simulink model "ADANISS_2R_Control"  (R2025b)
settings: Solver=ode45  StartTime=0  StopTime=40  MaxStep=0.0005  MinStep=1e-6  RelTol=1e-5  AbsTol=1e-7
libraries: slpidlib x2
settings Model: Creator=nicao  LastModifiedBy=nicao

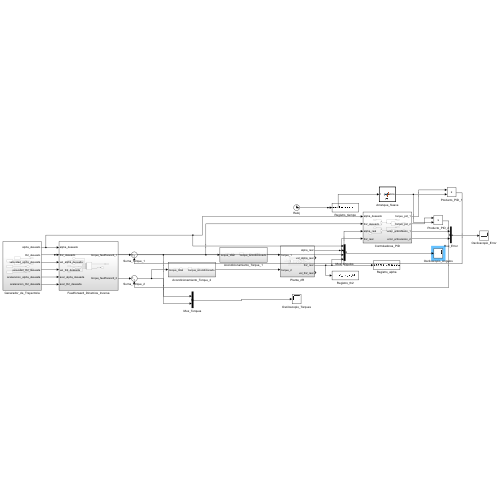
[thumbnail: Simulink's stored preview of the top-level diagram]
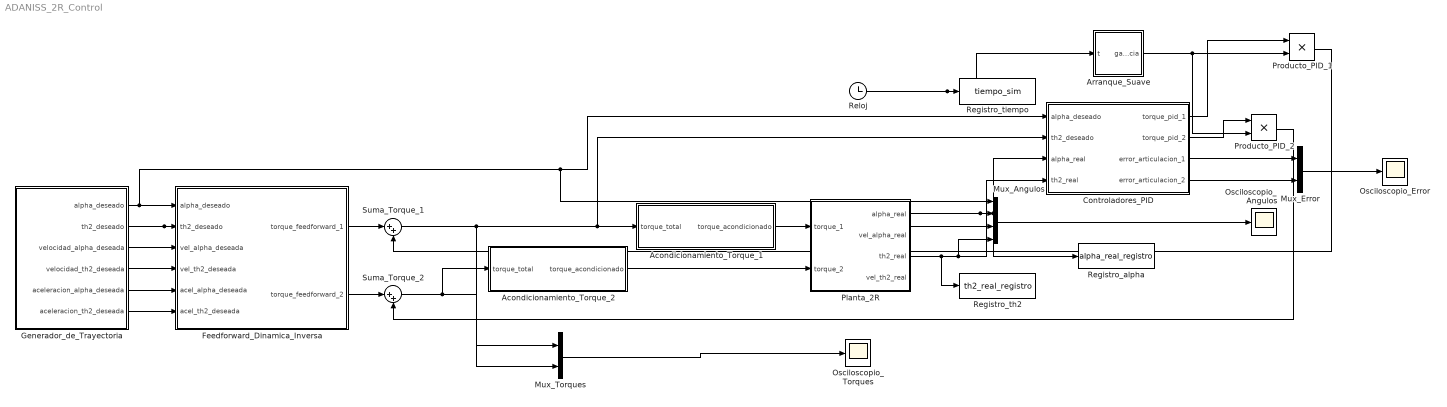
== system ADANISS_2R_Control ==
  Acondicionamiento_Torque_1 : Subsystem
  Acondicionamiento_Torque_2 : Subsystem
  Arranque_Suave : MATLAB Function  TreatAsAtomicUnit=on
  Controladores_PID : Subsystem
  Feedforward_Dinamica_Inversa : Subsystem
  Generador_de_Trayectoria : Subsystem
  Mux_Angulos : Mux
  Mux_Error : Mux  Inputs=2
  Mux_Torques : Mux  Inputs=2
  Osciloscopio_Angulos : Scope
      settings: ActiveDisplayYMinimum=-15.541303883024996  ActiveDisplayYMaximum=18.854538421738404
  Osciloscopio_Error : Scope
      settings: ActiveDisplayYMinimum=-0.62688226999815022  ActiveDisplayYMaximum=1.0560129058216277
  Osciloscopio_Torques : Scope
      settings: ActiveDisplayYMinimum=-3.9250000000000003  ActiveDisplayYMaximum=3.9250000000000003
  Planta_2R : Subsystem
  Producto_PID_1 : Product
  Producto_PID_2 : Product
  Registro_alpha : ToWorkspace  VariableName=alpha_real_registro
  Registro_th2 : ToWorkspace  VariableName=th2_real_registro
  Registro_tiempo : ToWorkspace  VariableName=tiempo_sim
  Reloj : Clock
  Suma_Torque_1 : Sum  Inputs=|++
  Suma_Torque_2 : Sum  Inputs=|++
  wires:
  Generador_de_Trayectoria/1(alpha_deseado) -> Mux_Angulos/1, Controladores_PID/1(alpha_deseado), Feedforward_Dinamica_Inversa/1(alpha_deseado)
  Generador_de_Trayectoria/2(th2_deseado) -> Mux_Angulos/3, Controladores_PID/2(th2_deseado), Feedforward_Dinamica_Inversa/2(th2_deseado)
  Generador_de_Trayectoria/3(velocidad_alpha_deseada) -> Feedforward_Dinamica_Inversa/3(vel_alpha_deseada)
  Generador_de_Trayectoria/4(velocidad_th2_deseada) -> Feedforward_Dinamica_Inversa/4(vel_th2_deseada)
  Generador_de_Trayectoria/5(aceleracion_alpha_deseada) -> Feedforward_Dinamica_Inversa/5(acel_alpha_deseada)
  Generador_de_Trayectoria/6(aceleracion_th2_deseada) -> Feedforward_Dinamica_Inversa/6(acel_th2_deseada)
  Planta_2R/1(alpha_real) -> Registro_alpha/1, Controladores_PID/3(alpha_real), Mux_Angulos/2
  Planta_2R/3(th2_real) -> Registro_th2/1, Mux_Angulos/4, Controladores_PID/4(th2_real)
  Suma_Torque_1/1 -> Mux_Torques/1, Acondicionamiento_Torque_1/1(torque_total)
  Suma_Torque_2/1 -> Acondicionamiento_Torque_2/1(torque_total), Mux_Torques/2
  Acondicionamiento_Torque_1/1(torque_acondicionado) -> Planta_2R/1(torque_1)
  Acondicionamiento_Torque_2/1(torque_acondicionado) -> Planta_2R/2(torque_2)
  Mux_Angulos/1 -> Osciloscopio_Angulos/1
  Mux_Torques/1 -> Osciloscopio_Torques/1
  Controladores_PID/3(error_articulacion_1) -> Mux_Error/1
  Controladores_PID/4(error_articulacion_2) -> Mux_Error/2
  Mux_Error/1 -> Osciloscopio_Error/1
  Reloj/1 -> Arranque_Suave/1(t), Registro_tiempo/1
  Arranque_Suave/1(ganancia) -> Producto_PID_2/2, Producto_PID_1/2
  Controladores_PID/1(torque_pid_1) -> Producto_PID_1/1
  Producto_PID_1/1 -> Suma_Torque_1/2
  Controladores_PID/2(torque_pid_2) -> Producto_PID_2/1
  Producto_PID_2/1 -> Suma_Torque_2/2
  Feedforward_Dinamica_Inversa/1(torque_feedforward_1) -> Suma_Torque_1/1
  Feedforward_Dinamica_Inversa/2(torque_feedforward_2) -> Suma_Torque_2/1

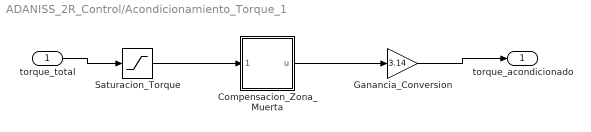
== system ADANISS_2R_Control/Acondicionamiento_Torque_1 ==
  torque_total : Inport
  Compensacion_Zona_Muerta : MATLAB Function  TreatAsAtomicUnit=on
  Ganancia_Conversion : Gain  Gain=3.14
  Saturacion_Torque : Saturate  UpperLimit=3.14  LowerLimit=-3.14
  torque_acondicionado : Outport
  wires:
  Saturacion_Torque/1 -> Compensacion_Zona_Muerta/1(tau_sat)
  Compensacion_Zona_Muerta/1(u) -> Ganancia_Conversion/1
  torque_total/1 -> Saturacion_Torque/1
  Ganancia_Conversion/1 -> torque_acondicionado/1

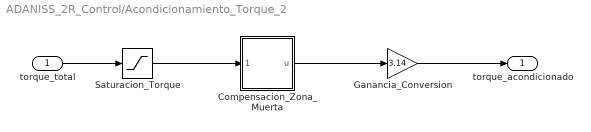
== system ADANISS_2R_Control/Acondicionamiento_Torque_2 ==
  torque_total : Inport
  Compensacion_Zona_Muerta : MATLAB Function  TreatAsAtomicUnit=on
  Ganancia_Conversion : Gain  Gain=3.14
  Saturacion_Torque : Saturate  UpperLimit=3.14  LowerLimit=-3.14
  torque_acondicionado : Outport
  wires:
  torque_total/1 -> Saturacion_Torque/1
  Saturacion_Torque/1 -> Compensacion_Zona_Muerta/1(tau_sat)
  Compensacion_Zona_Muerta/1(u) -> Ganancia_Conversion/1
  Ganancia_Conversion/1 -> torque_acondicionado/1

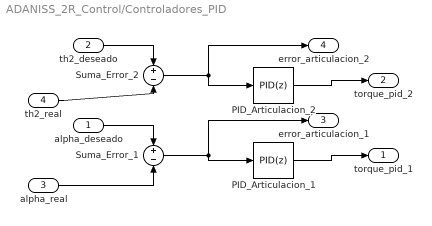
== system ADANISS_2R_Control/Controladores_PID ==
  alpha_deseado : Inport
  th2_deseado : Inport  Port=2
  alpha_real : Inport  Port=3
  th2_real : Inport  Port=4
  PID_Articulacion_1 : slpidlib/PID Controller  Controller=PID  Form=Parallel  TimeDomain=Discrete-time  UseExternalTs=off  SampleTime=0.001  IntegratorMethod=Forward Euler  FilterMethod=Forward Euler  ControllerParametersSource=internal  P=15  I=8  UseKiTs=off  D=1.2  UseExternalDerivativeSource=off  N=50  UseFilter=on  TunerSelectOption=Transfer Function Based (PID Tuner App)  InitialConditionSource=internal  InitialConditionForIntegrator=0  InitialConditionForFilter=0  DifferentiatorICPrevScaledInput=0  ExternalReset=none  TrackingMode=off  Kt=1  LimitOutput=on  SatLimitsSource=internal  UpperSaturationLimit=3.14  LowerSaturationLimit=-3.14  LinearizeAsGain=on  AntiWindupMode=clamping  Kb=1  LimitIntegrator=off  UpperIntegratorSaturationLimit=inf  LowerIntegratorSaturationLimit=-inf  POutMin=[]  POutMax=[]  IOutMin=[]  IOutMax=[]  DOutMin=[]  DOutMax=[]  NOutMin=[]  NOutMax=[]  SumOutMin=[]  SumOutMax=[]  SaturationOutMin=[]  SaturationOutMax=[]  PParamMin=[]  PParamMax=[]  IParamMin=[]  IParamMax=[]  DParamMin=[]  DParamMax=[]  NParamMin=[]  NParamMax=[]  KbParamMin=[]  KbParamMax=[]  KtParamMin=[]  KtParamMax=[]  KbOutMin=[]  KbOutMax=[]  KtOutMin=[]  KtOutMax=[]  IntegratorOutMin=[]  IntegratorOutMax=[]  FilterOutMin=[]  FilterOutMax=[]  SumI1OutMin=[]  SumI1OutMax=[]  SumI2OutMin=[]  SumI2OutMax=[]  SumI3OutMin=[]  SumI3OutMax=[]  SumI4OutMin=[]  SumI4OutMax=[]  SumDOutMin=[]  SumDOutMax=[]  DifferentiatorOutMin=[]  DifferentiatorOutMax=[]  FilterDiffOutCoefMin=[]  FilterDiffOutCoefMax=[]  ReciprocalOutMin=[]  ReciprocalOutMax=[]  SumDenOutMin=[]  SumDenOutMax=[]  SumNumOutMin=[]  SumNumOutMax=[]  DivideOutMin=[]  DivideOutMax=[]  UdiffTsProdOutMin=[]  UdiffTsProdOutMax=[]  NTsProdOutMin=[]  NTsProdOutMax=[]  UintegralTsProdOutMin=[]  UintegralTsProdOutMax=[]  UngainTsProdOutMin=[]  UngainTsProdOutMax=[]  ClampingZeroOutDataTypeStr=Inherit: Inherit via back propagation  ClampingZeroOutMin=[]  ClampingZeroOutMax=[]  FilterDenConstantOutDataTypeStr=Inherit: Inherit via back propagation  FilterDenConstantOutMin=[]  FilterDenConstantOutMax=[]  PCopyOutDataTypeStr=Inherit: Inherit via back propagation  PCopyOutMin=[]  PCopyOutMax=[]  NCopyOutDataTypeStr=Inherit: Inherit via back propagation  NCopyOutMin=[]  NCopyOutMax=[]  IntegratorContinuousStateAttributes=''  IntegratorStateMustResolveToSignalObject=off  IntegratorRTWStateStorageClass=Auto  FilterContinuousStateAttributes=''  FilterStateMustResolveToSignalObject=off  FilterRTWStateStorageClass=Auto  ParallelPVariant=InternalParameters  IdealPVariant=Disabled  IVariant=InternalParameters  DVariant=InternalParameters  IntegratorVariant=Discrete  SatVariant=Enabled  AWVariant=DiscClampingParallel  PCopyVariant=Disabled  TRVariant=Disabled  FdbkBlocksVariant=Forward  IdealPFdbkVariant=Disabled  SatFdbkVariant=Disabled  DerivativeFilterVariant=ForwardEulerFilter  NVariant=InternalParameters  NCopyVariant=Disabled  FilterICVariant=InternalICsFilter  IntegratorICVariant=InternalICs  ExternalResetVariant=Disabled  TRSumVariant=Passthrough  SumFdbkVariant=Disabled  SumVariant=Sum_PID  TsampFilterVariant=InternalTs  TsampNgainVariant=Passthrough  TsampIntegralVariant=Disabled_SignalSpec  ExternalSaturationOutDataTypeStr=Inherit: Same as second input  DerivativeSourceVariant=ErrorSignal  PreIntVariant=InternalPreInt
  PID_Articulacion_2 : slpidlib/PID Controller  Controller=PID  Form=Parallel  TimeDomain=Discrete-time  UseExternalTs=off  SampleTime=0.001  IntegratorMethod=Forward Euler  FilterMethod=Forward Euler  ControllerParametersSource=internal  P=15  I=8  UseKiTs=off  D=1.2  UseExternalDerivativeSource=off  N=50  UseFilter=on  TunerSelectOption=Transfer Function Based (PID Tuner App)  InitialConditionSource=internal  InitialConditionForIntegrator=0  InitialConditionForFilter=0  DifferentiatorICPrevScaledInput=0  ExternalReset=none  TrackingMode=off  Kt=1  LimitOutput=on  SatLimitsSource=internal  UpperSaturationLimit=3.14  LowerSaturationLimit=-3.14  LinearizeAsGain=on  AntiWindupMode=clamping  Kb=1  LimitIntegrator=off  UpperIntegratorSaturationLimit=inf  LowerIntegratorSaturationLimit=-inf  POutMin=[]  POutMax=[]  IOutMin=[]  IOutMax=[]  DOutMin=[]  DOutMax=[]  NOutMin=[]  NOutMax=[]  SumOutMin=[]  SumOutMax=[]  SaturationOutMin=[]  SaturationOutMax=[]  PParamMin=[]  PParamMax=[]  IParamMin=[]  IParamMax=[]  DParamMin=[]  DParamMax=[]  NParamMin=[]  NParamMax=[]  KbParamMin=[]  KbParamMax=[]  KtParamMin=[]  KtParamMax=[]  KbOutMin=[]  KbOutMax=[]  KtOutMin=[]  KtOutMax=[]  IntegratorOutMin=[]  IntegratorOutMax=[]  FilterOutMin=[]  FilterOutMax=[]  SumI1OutMin=[]  SumI1OutMax=[]  SumI2OutMin=[]  SumI2OutMax=[]  SumI3OutMin=[]  SumI3OutMax=[]  SumI4OutMin=[]  SumI4OutMax=[]  SumDOutMin=[]  SumDOutMax=[]  DifferentiatorOutMin=[]  DifferentiatorOutMax=[]  FilterDiffOutCoefMin=[]  FilterDiffOutCoefMax=[]  ReciprocalOutMin=[]  ReciprocalOutMax=[]  SumDenOutMin=[]  SumDenOutMax=[]  SumNumOutMin=[]  SumNumOutMax=[]  DivideOutMin=[]  DivideOutMax=[]  UdiffTsProdOutMin=[]  UdiffTsProdOutMax=[]  NTsProdOutMin=[]  NTsProdOutMax=[]  UintegralTsProdOutMin=[]  UintegralTsProdOutMax=[]  UngainTsProdOutMin=[]  UngainTsProdOutMax=[]  ClampingZeroOutDataTypeStr=Inherit: Inherit via back propagation  ClampingZeroOutMin=[]  ClampingZeroOutMax=[]  FilterDenConstantOutDataTypeStr=Inherit: Inherit via back propagation  FilterDenConstantOutMin=[]  FilterDenConstantOutMax=[]  PCopyOutDataTypeStr=Inherit: Inherit via back propagation  PCopyOutMin=[]  PCopyOutMax=[]  NCopyOutDataTypeStr=Inherit: Inherit via back propagation  NCopyOutMin=[]  NCopyOutMax=[]  IntegratorContinuousStateAttributes=''  IntegratorStateMustResolveToSignalObject=off  IntegratorRTWStateStorageClass=Auto  FilterContinuousStateAttributes=''  FilterStateMustResolveToSignalObject=off  FilterRTWStateStorageClass=Auto  ParallelPVariant=InternalParameters  IdealPVariant=Disabled  IVariant=InternalParameters  DVariant=InternalParameters  IntegratorVariant=Discrete  SatVariant=Enabled  AWVariant=DiscClampingParallel  PCopyVariant=Disabled  TRVariant=Disabled  FdbkBlocksVariant=Forward  IdealPFdbkVariant=Disabled  SatFdbkVariant=Disabled  DerivativeFilterVariant=ForwardEulerFilter  NVariant=InternalParameters  NCopyVariant=Disabled  FilterICVariant=InternalICsFilter  IntegratorICVariant=InternalICs  ExternalResetVariant=Disabled  TRSumVariant=Passthrough  SumFdbkVariant=Disabled  SumVariant=Sum_PID  TsampFilterVariant=InternalTs  TsampNgainVariant=Passthrough  TsampIntegralVariant=Disabled_SignalSpec  ExternalSaturationOutDataTypeStr=Inherit: Same as second input  DerivativeSourceVariant=ErrorSignal  PreIntVariant=InternalPreInt
  Suma_Error_1 : Sum  Inputs=+-
  Suma_Error_2 : Sum  Inputs=+-
  torque_pid_1 : Outport
  torque_pid_2 : Outport  Port=2
  error_articulacion_1 : Outport  Port=3
  error_articulacion_2 : Outport  Port=4
  wires:
  alpha_deseado/1 -> Suma_Error_1/1
  alpha_real/1 -> Suma_Error_1/2
  th2_deseado/1 -> Suma_Error_2/1
  th2_real/1 -> Suma_Error_2/2
  Suma_Error_1/1 -> PID_Articulacion_1/1, error_articulacion_1/1
  Suma_Error_2/1 -> PID_Articulacion_2/1, error_articulacion_2/1
  PID_Articulacion_1/1 -> torque_pid_1/1
  PID_Articulacion_2/1 -> torque_pid_2/1

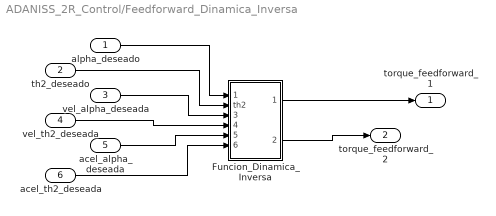
== system ADANISS_2R_Control/Feedforward_Dinamica_Inversa ==
  alpha_deseado : Inport
  th2_deseado : Inport  Port=2
  vel_alpha_deseada : Inport  Port=3
  vel_th2_deseada : Inport  Port=4
  acel_alpha_deseada : Inport  Port=5
  acel_th2_deseada : Inport  Port=6
  Funcion_Dinamica_Inversa : MATLAB Function  TreatAsAtomicUnit=on
  torque_feedforward_1 : Outport
  torque_feedforward_2 : Outport  Port=2
  wires:
  alpha_deseado/1 -> Funcion_Dinamica_Inversa/1(alpha)
  Funcion_Dinamica_Inversa/1(tau_ff1) -> torque_feedforward_1/1
  th2_deseado/1 -> Funcion_Dinamica_Inversa/2(th2)
  vel_alpha_deseada/1 -> Funcion_Dinamica_Inversa/3(dalpha)
  vel_th2_deseada/1 -> Funcion_Dinamica_Inversa/4(dth2)
  acel_alpha_deseada/1 -> Funcion_Dinamica_Inversa/5(d2alpha)
  acel_th2_deseada/1 -> Funcion_Dinamica_Inversa/6(d2th2)
  Funcion_Dinamica_Inversa/2(tau_ff2) -> torque_feedforward_2/1

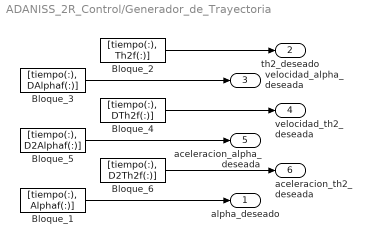
== system ADANISS_2R_Control/Generador_de_Trayectoria ==
  Bloque_1 : FromWorkspace  VariableName=[tiempo(:), Alphaf(:)]
  Bloque_2 : FromWorkspace  VariableName=[tiempo(:), Th2f(:)]
  Bloque_3 : FromWorkspace  VariableName=[tiempo(:), DAlphaf(:)]
  Bloque_4 : FromWorkspace  VariableName=[tiempo(:), DTh2f(:)]
  Bloque_5 : FromWorkspace  VariableName=[tiempo(:), D2Alphaf(:)]
  Bloque_6 : FromWorkspace  VariableName=[tiempo(:), D2Th2f(:)]
  alpha_deseado : Outport
  th2_deseado : Outport  Port=2
  velocidad_alpha_deseada : Outport  Port=3
  velocidad_th2_deseada : Outport  Port=4
  aceleracion_alpha_deseada : Outport  Port=5
  aceleracion_th2_deseada : Outport  Port=6
  wires:
  Bloque_1/1 -> alpha_deseado/1
  Bloque_2/1 -> th2_deseado/1
  Bloque_3/1 -> velocidad_alpha_deseada/1
  Bloque_4/1 -> velocidad_th2_deseada/1
  Bloque_5/1 -> aceleracion_alpha_deseada/1
  Bloque_6/1 -> aceleracion_th2_deseada/1

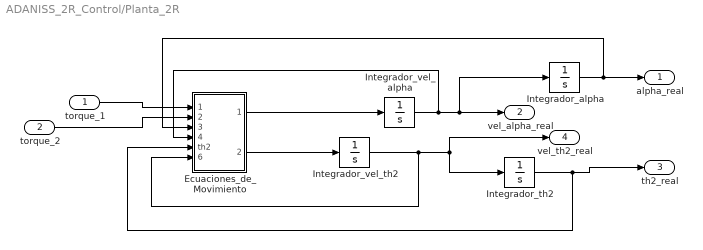
== system ADANISS_2R_Control/Planta_2R ==
  torque_1 : Inport
  torque_2 : Inport  Port=2
  Ecuaciones_de_Movimiento : MATLAB Function  TreatAsAtomicUnit=on
  Integrador_alpha : Integrator
  Integrador_th2 : Integrator  InitialCondition=3.141592653589793
  Integrador_vel_alpha : Integrator  InitialCondition=0.0004502450016226697
  Integrador_vel_th2 : Integrator  InitialCondition=-0.0003575475012871365
  alpha_real : Outport
  vel_alpha_real : Outport  Port=2
  th2_real : Outport  Port=3
  vel_th2_real : Outport  Port=4
  wires:
  torque_1/1 -> Ecuaciones_de_Movimiento/1(tau1)
  Ecuaciones_de_Movimiento/1(ddq1) -> Integrador_vel_alpha/1
  Integrador_vel_alpha/1 -> vel_alpha_real/1, Integrador_alpha/1, Ecuaciones_de_Movimiento/4(dalpha)
  Integrador_vel_th2/1 -> vel_th2_real/1, Integrador_th2/1, Ecuaciones_de_Movimiento/6(dth2)
  Integrador_alpha/1 -> Ecuaciones_de_Movimiento/3(alpha), alpha_real/1
  Integrador_th2/1 -> Ecuaciones_de_Movimiento/5(th2), th2_real/1
  torque_2/1 -> Ecuaciones_de_Movimiento/2(tau2)
  Ecuaciones_de_Movimiento/2(ddq2) -> Integrador_vel_th2/1

== matlab function ADANISS_2R_Control/Acondicionamiento_Torque_1/Compensacion_Zona_Muerta ==
  data: tau_sat input; u output
function u = fcn(tau_sat)
  % Compensa la fricción interna de los engranajes (zona muerta).
  % Si el torque es muy bajo, el motor no se mueve.
  zona_muerta = 1.5/12;   % El 12.5% de la potencia es para vencer el roce
  tau_max     = 3.14;     % Torque máximo de bloqueo
  if abs(tau_sat) > 0.005
    % Si el torque es suficiente, lo escalamos para saltar la zona muerta
    u = sign(tau_sat)*zona_muerta + (1 - zona_muerta)*(tau_sat/tau_max);
  else
    u = 0; % Si es casi cero, no enviamos señal al motor
  end
end

== matlab function ADANISS_2R_Control/Feedforward_Dinamica_Inversa/Funcion_Dinamica_Inversa ==
  data: alpha input; tau_ff1 output; th2 input; dalpha input; dth2 input; d2alpha input; d2th2 input; tau_ff2 output
function [tau_ff1, tau_ff2] = fcn(alpha, th2, dalpha, dth2, d2alpha, d2th2)
  tau_ff1 = 0; tau_ff2 = 0;
end

== matlab function ADANISS_2R_Control/Acondicionamiento_Torque_2/Compensacion_Zona_Muerta ==
  data: tau_sat input; u output
function u = fcn(tau_sat)
  % Compensa la fricción interna de los engranajes (zona muerta).
  % Si el torque es muy bajo, el motor no se mueve.
  zona_muerta = 1.5/12;   % El 12.5% de la potencia es para vencer el roce
  tau_max     = 3.14;     % Torque máximo de bloqueo
  if abs(tau_sat) > 0.005
    % Si el torque es suficiente, lo escalamos para saltar la zona muerta
    u = sign(tau_sat)*zona_muerta + (1 - zona_muerta)*(tau_sat/tau_max);
  else
    u = 0; % Si es casi cero, no enviamos señal al motor
  end
end

== matlab function ADANISS_2R_Control/Planta_2R/Ecuaciones_de_Movimiento ==
  data: tau1 input; ddq1 output; tau2 input; alpha input; dalpha input; th2 input; dth2 input; ddq2 output
function [ddq1, ddq2] = dinamica_planta(tau1, tau2, alpha, dalpha, th2, dth2)
  % 1. PARÁMETROS FÍSICOS DEL ROBOT
  m1=0.1; m2=0.1; L1=0.235; L2=0.235; lc1=3*L1/4; lc2=3*L2/4;
  Iz1=(1/12)*m1*(0.03^2+0.01^2); % Inercia rotacional eslabón 1
  Iz2=(1/12)*m2*(0.03^2+0.01^2); % Inercia rotacional eslabón 2
  gr=9.8; % Gravedad

  % 2. CINEMÁTICA Y GEOMETRÍA
  beta  = -(pi - th2); % Ángulo relativo del codo
  c2    = cos(beta); s2 = sin(beta); % Seno y coseno de beta
  c12   = cos(alpha+beta); c1 = cos(alpha); % Ángulos compuestos

  % 3. CÁLCULO DE MATRICES DINÁMICAS (M, C, G)
  M11   = m1*lc1^2+Iz1+m2*L1^2+m2*lc2^2+Iz2+2*m2*L1*lc2*c2; % Matriz de masa (Inercia total)
  M12   = m2*lc2^2+Iz2+m2*L1*lc2*c2;
  M22   = m2*lc2^2+Iz2;
  E     = 2*m2*L1*lc2*s2; % Término de Coriolis
  N_c   = -m2*L1*lc2*s2;
  C1    = E*dalpha*dth2 + E*dth2^2; % Fuerzas centrífugas 1
  C2    = N_c*dalpha*dth2 + m2*L1*lc2*s2*dalpha^2; % Fuerzas centrífugas 2
  G1    = gr*((m1*lc1+m2*L1)*c1 + m2*lc2*c12); % Gravedad en articulación 1
  G2    = gr*(m2*lc2*c12); % Gravedad en articulación 2

  % 4. RESOLVER SISTEMA: ddq = inv(M) * (tau - C - G)
  det_M = M11*M22 - M12^2; % Determinante para la inversión
  res1 = tau1 - C1 - G1; % Torque neto 1
  res2 = tau2 - C2 - G2; % Torque neto 2
  ddq1 = ( M22*res1 - M12*res2) / det_M; % Aceleración angular 1
  ddq2 = (-M12*res1 + M11*res2) / det_M; % Aceleración angular 2
end

== matlab function ADANISS_2R_Control/Arranque_Suave ==
  data: t input; ganancia output
function ganancia = fcn(t)
  % Este bloque suaviza la fuerza del PID al inicio
  % para evitar que el robot salte bruscamente.
  t_ramp = 8.0; % Tiempo que dura la rampa (8 segundos)
  if t < t_ramp
    u = t / t_ramp; % Variable normalizada de 0 a 1
    % Función polinómica S-Curve (suave al inicio y al final)
    ganancia = 10*u^3 - 15*u^4 + 6*u^5;
  else
    ganancia = 1.0; % Ganancia total después de la rampa
  end
end
